simulink model "pole_simulink"  (R2021b)
settings: Solver=VariableStepAuto  StartTime=0.0  StopTime=10  RelTol=1e-3
values from neighbouring files (symbols this model uses):
  A = [0, 0, 0, 1, 0, 0 ... (first row only)    [basic_data.m]    (also in basic_data.mat = [0 0 0 0 -22.4688936865 5 0 0 0 6.5 19.3959496459 -3.6 ... (; lqr.mat = [0 0 0 0 -22.4688936865 5 0 0 0 6.5 19.3959496459 -3.6 ... ()
  B = [0, 0 ... (first row only)    [basic_data.m]    (also in basic_data.mat = [0  0; 0  0; 0  0; 27  11.2; 6.06660129535  -1.63757677119; ; lqr.mat = [0  0; 0  0; 0  0; 27  11.2; 6.06660129535  -1.63757677119; )
  C = [1, 0, 0, 0, 0, 0 ... (first row only)    [basic_data.m]    (also in basic_data.mat = [1 0 0 0 1 0 0 0 1 0 0 0 ... (18 elements, 3x6)]; lqr.mat = [1 0 0 0 1 0 0 0 1 0 0 0 ... (18 elements, 3x6)])
  K_build = lqr(A,B,Q,R)    [LQR.m]    (also in lqr.mat = [-254.853126295  165.420589599  161.115517612  -14.47290047 ; pole_placement.m = place(A,B,p))
settings Model: Creator=asus  LastModifiedBy=asus

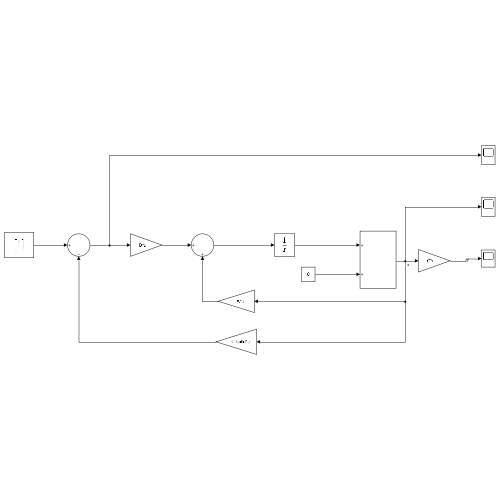
[thumbnail: Simulink's stored preview of the top-level diagram]
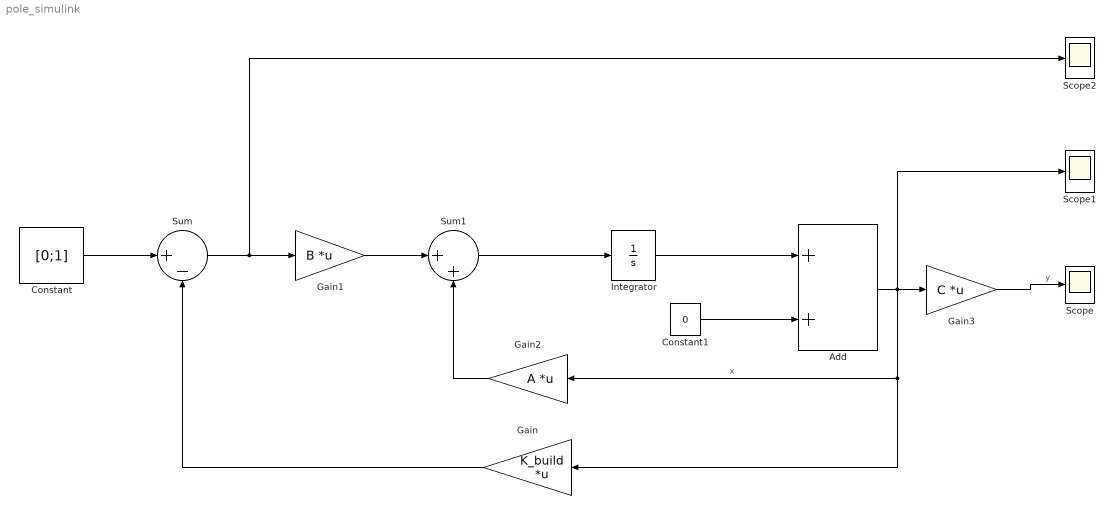
== system pole_simulink ==
  Add : Sum
  Constant : Constant  Value=[0;1]  VectorParams1D=off
  Constant1 : Constant  Value=0  VectorParams1D=off
  Gain : Gain  Gain=K_build  Multiplication=Matrix(K*u)
  Gain1 : Gain  Gain=B  Multiplication=Matrix(K*u)
  Gain2 : Gain  Gain=A  Multiplication=Matrix(K*u)
  Gain3 : Gain  Gain=C  Multiplication=Matrix(K*u)
  Integrator : Integrator
  Scope : Scope
  Scope1 : Scope
  Scope2 : Scope
  Sum : Sum  Inputs=|+-
  Sum1 : Sum  Inputs=|++
  wires:
  Integrator/1 -> Add/1
  Gain/1 -> Sum/2
  Sum1/1 -> Integrator/1
  Sum/1 -> Scope2/1, Gain1/1
  Gain1/1 -> Sum1/1
  Gain2/1 -> Sum1/2
  Constant/1 -> Sum/1
  Gain3/1 -> Scope/1  "y"
  Add/1 -> Scope1/1, Gain/1, Gain2/1, Gain3/1  "x"
  Constant1/1 -> Add/2
